simulink model "CSTR (1) (1)"  (R2024a)
settings: Solver=VariableStepAuto  StartTime=0.0  StopTime=10.0  RelTol=1e-3

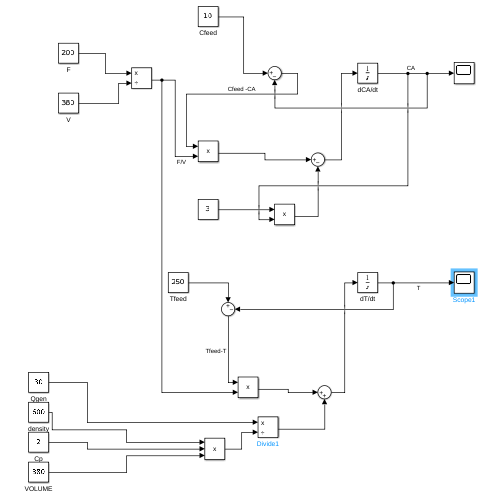
[thumbnail: Simulink's stored preview of the top-level diagram]
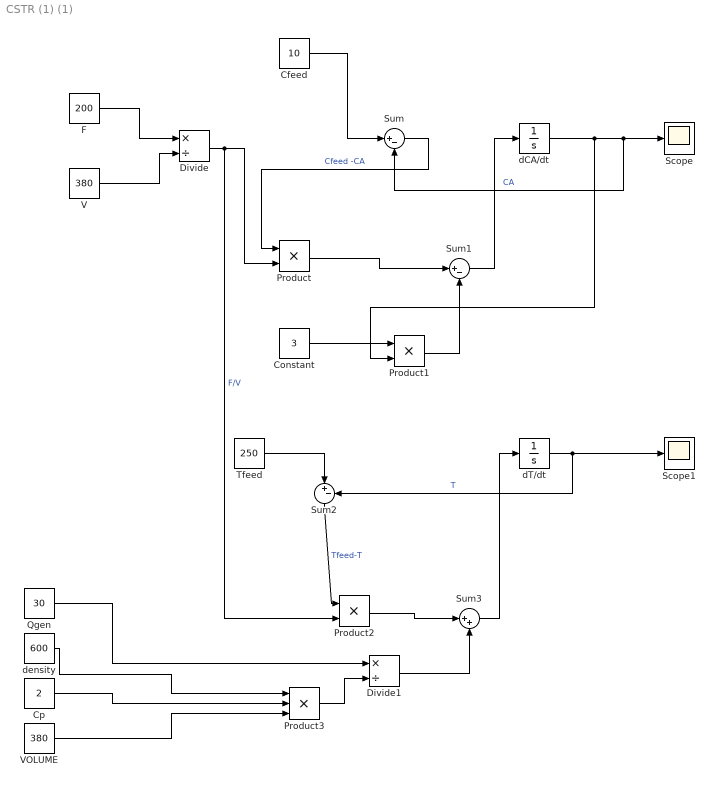
== system CSTR (1) (1) ==
  Cfeed : Constant  Value=10
  Constant : Constant  Value=3
  Cp : Constant  Value=2
  Divide : Product  Inputs=*/
  Divide1 : Product  Inputs=*/
  F : Constant  Value=200  VectorParams1D=off
  Product : Product
  Product1 : Product
  Product2 : Product
  Product3 : Product  Inputs=3
  Qgen : Constant  Value=30
  Scope : Scope
  Scope1 : Scope
  Sum : Sum  Inputs=|+-
  Sum1 : Sum  Inputs=|+-
  Sum2 : Sum  Inputs=|+-
  Sum3 : Sum  Inputs=|++
  Tfeed : Constant  Value=250
  V : Constant  Value=380
  VOLUME : Constant  Value=380
  dCA/dt : Integrator
  dT/dt : Integrator
  density : Constant  Value=600
  wires:
  F/1 -> Divide/1
  V/1 -> Divide/2
  dCA/dt/1 -> Scope/1, Sum/2, Product1/2  "CA"
  Cfeed/1 -> Sum/1
  Divide/1 -> Product2/2, Product/2  "F/V"
  Sum/1 -> Product/1  "Cfeed -CA"
  Sum1/1 -> dCA/dt/1
  Product/1 -> Sum1/1
  Product1/1 -> Sum1/2
  Constant/1 -> Product1/1
  Tfeed/1 -> Sum2/1
  dT/dt/1 -> Sum2/2, Scope1/1  "T"
  Sum2/1 -> Product2/1  "Tfeed-T"
  density/1 -> Product3/1
  Cp/1 -> Product3/2
  VOLUME/1 -> Product3/3
  Product3/1 -> Divide1/2
  Qgen/1 -> Divide1/1
  Product2/1 -> Sum3/1
  Divide1/1 -> Sum3/2
  Sum3/1 -> dT/dt/1
